simulink model "Reg_Obs"  (R2017b)
settings: Solver=VariableStepAuto  StartTime=0.0  StopTime=5.0  RelTol=1e-3
values from neighbouring files (symbols this model uses):
  A = [c1 c2  0    c3      0 ... (first row only)    [Regul_Luenbergh.m]    (also in Regul_Luenbergh2.m; Regul_Modal.m; Regul_Modal2.m; Regul_Optim.m)
  B = [0; 0; 0; 0; iv/Tcn]    [Regul_Luenbergh.m]    (also in Regul_Luenbergh2.m; Regul_Modal.m; Regul_Modal2.m; Regul_Optim.m)
  C = [0 1 0 0 0]    [Regul_Luenbergh.m]    (also in Regul_Luenbergh2.m; Regul_Modal.m; Regul_Modal2.m; Regul_Optim.m)
  k = Q'\(a-az)    [Regul_Luenbergh.m]    (also in Regul_Modal.m = Q'\(a-az),; Regul_Modal2.m)
  L = -((T'*Sn')^(-1))*(az-az_nab)    [Regul_Luenbergh.m]
settings Model: Creator=ASUS_302  LastModifiedBy=ASUS_302

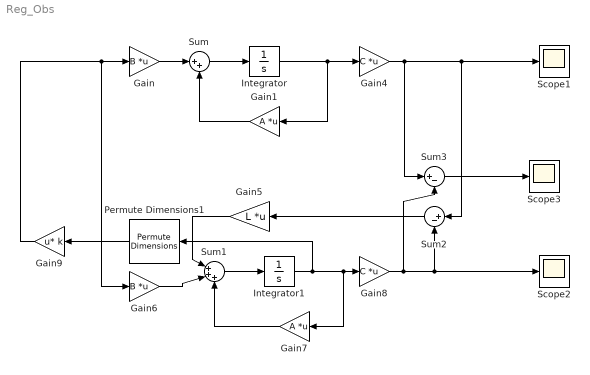
== system Reg_Obs ==
  Gain : Gain  Gain=B  Multiplication=Matrix(K*u)
  Gain1 : Gain  Gain=A  Multiplication=Matrix(K*u)
  Gain4 : Gain  Gain=C  Multiplication=Matrix(K*u)
  Gain5 : Gain  Gain=L  Multiplication=Matrix(K*u)
  Gain6 : Gain  Gain=B  Multiplication=Matrix(K*u)
  Gain7 : Gain  Gain=A  Multiplication=Matrix(K*u)
  Gain8 : Gain  Gain=C  Multiplication=Matrix(K*u)
  Gain9 : Gain  Gain=k  Multiplication=Matrix(u*K)
  Integrator : Integrator  InitialCondition=[1;1;1;1;1]
  Integrator1 : Integrator  InitialCondition=[0;0;0;0;0]
  Permute Dimensions1 : PermuteDimensions
  Scope1 : Scope
  Scope2 : Scope
  Scope3 : Scope
  Sum : Sum  Inputs=|++
  Sum1 : Sum  Inputs=|+++
  Sum2 : Sum  Inputs=|+-
  Sum3 : Sum  Inputs=|+-
  wires:
  Sum/1 -> Integrator/1
  Integrator/1 -> Gain1/1, Gain4/1
  Gain4/1 -> Sum3/1, Sum2/1, Scope1/1
  Gain5/1 -> Sum1/1
  Gain6/1 -> Sum1/2
  Gain7/1 -> Sum1/3
  Sum1/1 -> Integrator1/1
  Integrator1/1 -> Permute Dimensions1/1, Gain7/1, Gain8/1
  Gain8/1 -> Sum3/2, Scope2/1, Sum2/2
  Gain9/1 -> Gain6/1, Gain/1
  Permute Dimensions1/1 -> Gain9/1
  Gain/1 -> Sum/1
  Gain1/1 -> Sum/2
  Sum2/1 -> Gain5/1
  Sum3/1 -> Scope3/1
